simulink model "SIXTH"  (R2020b)
settings: Solver=FixedStepDiscrete  StartTime=0.0  StopTime=20.0  FixedStep=0.001  RelTol=1e-3
PreLoadFcn:
  | a0=1;
  | a1=2;
  | a2=-3;
  | a3=-4;
  | a4=5;
PostLoadFcn:
  | a0=1;
  | a1=2;
  | a2=-3;
  | a3=-4;
  | a4=5;
settings Model: Creator=priyaD  LastModifiedBy=priyaD
settings DataIOCC: SaveFormat=Array  DSMLogging=off

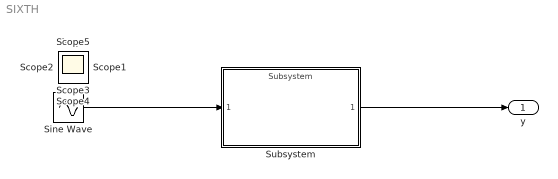
== system SIXTH ==
  Sine Wave : Sin  SampleTime=0
  Subsystem : ModelReference  ModelNameDialog=Subsystem  ModelReferenceVersion=1.3
  y : Outport
  Scope{,1..5} (6 alike) : Scope
  wires:
  Sine Wave/1 -> Subsystem/1
  Subsystem/1 -> y/1
